simulink model "model"  (R2021b)
settings: Solver=FixedStepAuto  StartTime=0.0  StopTime=inf  FixedStep=t_s  RelTol=1e-3
values from neighbouring files (symbols this model uses):
  Amp = 1    [par.m]
  Bias = 1    [par.m]
  Freq = 1    [par.m]
  Phase = 3    [par.m]
  t_s = 0.1    [par.m]
libraries: instrumentseriallib x3
settings Model: Creator=16970  LastModifiedBy=16970

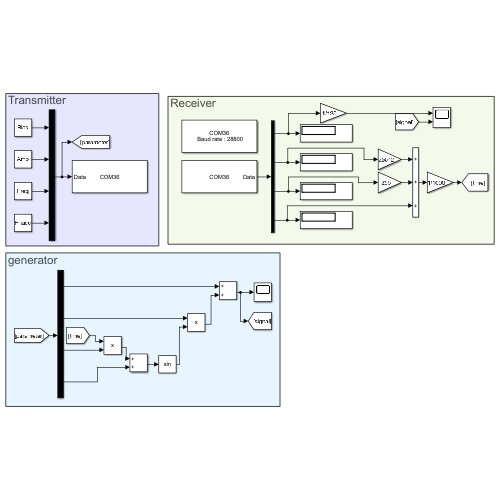
[thumbnail: Simulink's stored preview of the top-level diagram]
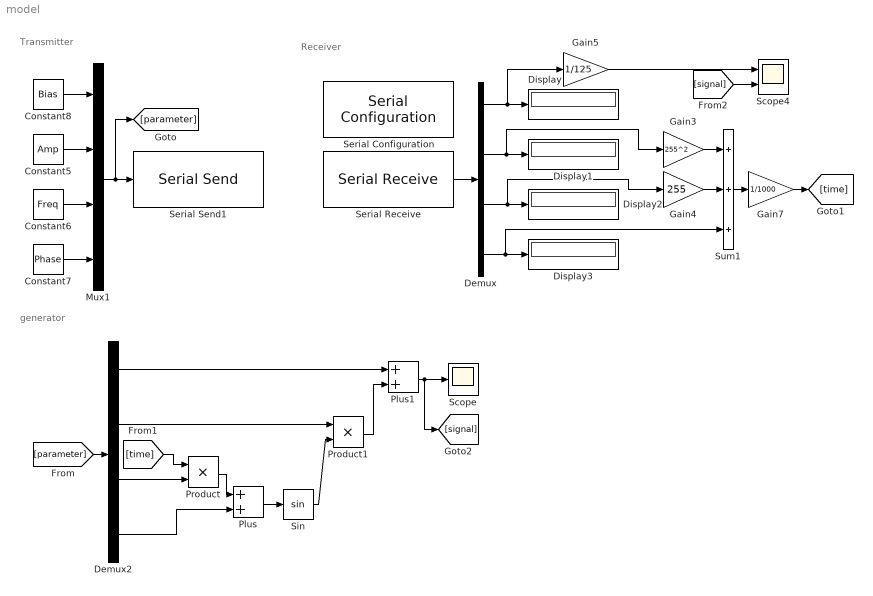
== system model ==
  note: generator
  note: Receiver
  note: Transmitter
  Constant5 : Constant  Value=Amp  OutDataTypeStr=uint8  SampleTime=t_s
  Constant6 : Constant  Value=Freq  OutDataTypeStr=uint8  SampleTime=t_s
  Constant7 : Constant  Value=Phase  OutDataTypeStr=uint8  SampleTime=t_s
  Constant8 : Constant  Value=Bias  OutDataTypeStr=uint8  SampleTime=t_s
  Demux : Demux
  Demux2 : Demux
  Display{,1..3} (4 alike) : Display
  Gain3 : Gain  Gain=255^2
  Gain4 : Gain  Gain=255
  Gain5 : Gain  Gain=1/125
  Gain7 : Gain  Gain=1/1000
  Mux1 : Mux
  Plus : Sum  OutDataTypeStr=double  LockScale=on
  Plus1 : Sum
  Product : Product
  Product1 : Product
  Scope : Scope
  Scope4 : Scope  NumInputPorts=2
  Serial Configuration : instrumentseriallib/Serial Configuration  Priority=-200000  Port=COM36  ComPort=COM36  BaudRate=28800  DataBits=8  Parity=none  StopBits=1  ByteOrder=little-endian  FlowControl=none  Timeout=100  SimulateUsing=Interpreted execution  BlockInModel=on
  Serial Receive : instrumentseriallib/Serial Receive  Priority=1  Port=COM36  ComPort=COM36  DataType=uint8  SaveDataType=uint8  ToggleHeader=on  Header=['H']  ToggleTerminator=on  Terminator=Custom terminator  CustomTerminator=['T']  ToggleDataSize=on  DataSize=[1 4]  EnableBlockingMode=on  ActionDataUnavailable=Error  ActionWhenDataUnavailable=Error  CustomValue=0  SampleTime=t_s  SimulateUsing=Interpreted execution  BlockInModel=on
  Serial Send1 : instrumentseriallib/Serial Send  Priority=1  Port=COM36  ComPort=COM36  Header=[]  Terminator=<none>  CustomTerminator=['T']  EnableBlockingMode=on  SimulateUsing=Interpreted execution  BlockInModel=on
  Sin : Trigonometry
  Sum1 : Sum  Inputs=+++
  wires:
  Serial Receive/1 -> Demux/1
  Demux/1 -> Gain5/1, Display/1
  Demux/2 -> Gain3/1, Display1/1
  Demux/3 -> Gain4/1, Display2/1
  Demux/4 -> Sum1/3, Display3/1
  Constant5/1 -> Mux1/2
  Constant8/1 -> Mux1/1
  Constant6/1 -> Mux1/3
  Demux2/4 -> Plus/2
  Demux2/3 -> Product/2
  Demux2/2 -> Product1/1
  Product/1 -> Plus/1
  Plus/1 -> Sin/1
  Sin/1 -> Product1/2
  Product1/1 -> Plus1/2
  Demux2/1 -> Plus1/1
  Plus1/1 -> Scope/1, [signal]
  Gain3/1 -> Sum1/1
  Gain4/1 -> Sum1/2
  Gain5/1 -> Scope4/1
  Mux1/1 -> [parameter], Serial Send1/1
  Constant7/1 -> Mux1/4
  [parameter] -> Demux2/1
  Sum1/1 -> Gain7/1
  Gain7/1 -> [time]
  [time] -> Product/1
  [signal] -> Scope4/2
